simulink model "single_pend"  (R2019b)
settings: Solver=VariableStepAuto  StartTime=0.0  StopTime=20  RelTol=1e-3
values from neighbouring files (symbols this model uses):
  b = 200    [single_pend_runner.m]
  eta = 30.0    (= 30)    [single_pend_runner.m]
  g = 9.81    [G.m]    (also in connect_pend_runner.m = -9.81; run.m; single_pend_runner.m = -9.81)
  Kd = 50    [anujay_single_pendulum_same.m]    (also in connect_pend_runner.m; double_pend_setup.m = [50,0;0,50]; single_pend_runner.m = 500)
  Kp = 500    [single_pend_runner.m]
  l2 = l1    (= 1)    [connect_pend_runner.m]    (also in single_pend_runner.m = 3)
  lambda = 1.0    (= 1)    [single_pend_runner.m]
  m2 = 1.0 + m1    (= 2)    [connect_pend.m]    (also in connect_pend_runner.m; single_pend_runner.m = 10)
libraries: robotcorelib x1, simulink x1
settings Model: Creator=nathanielgoldfarb  LastModifiedBy=nathanielgoldfarb
settings SolverCC: ZeroCrossAlgorithm=Adaptive
settings DebuggingCC: IgnoredZcDiagnostic=none

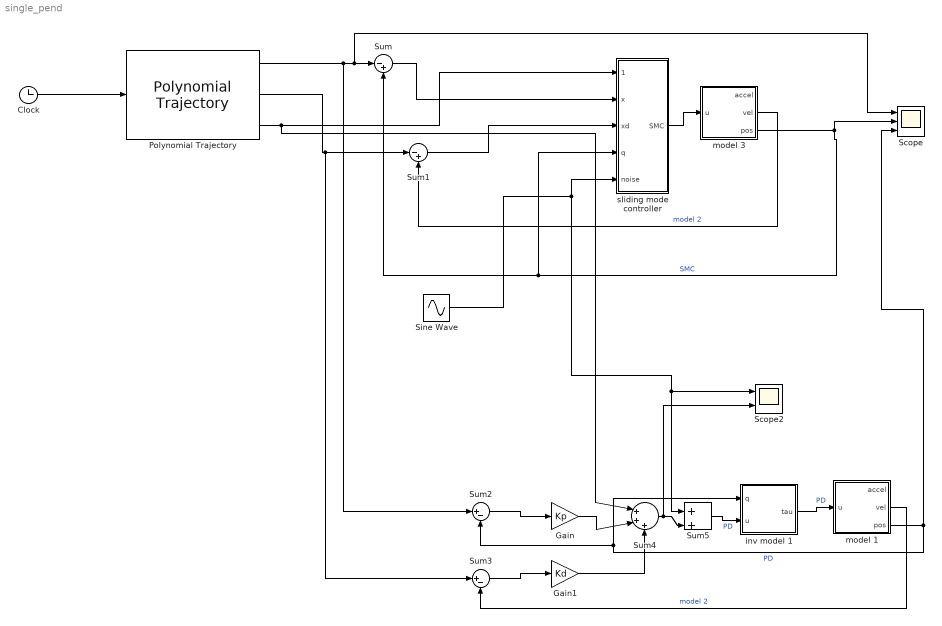
== system single_pend ==
  Clock : Clock
  Gain : Gain  Gain=Kp
  Gain1 : Gain  Gain=Kd
  Polynomial Trajectory : robotcorelib/Polynomial Trajectory  WaypointSource=Internal  Waypoints="[0  -pi ]"  TimePoints="[ 0,  5 ]"  TimeInterval=[ 1, 4 ]  Method=Cubic Polynomial  ParameterSource=Internal  VelocityBoundaryCondition=zeros( 1, 2 )  AccelerationBoundaryCondition=zeros( 2, 5 )  SimulateUsing=Interpreted execution
      settings: SourceProductName=Robotics System Toolbox  SourceProductBaseCode=RO
  Scope : Scope  NumInputPorts=3
  Scope2 : Scope  NumInputPorts=2
  Sine Wave : Sin  Amplitude=5  Frequency=50  SampleTime=0
  Sum : Sum  Inputs=|-+
  Sum1 : Sum  Inputs=|-+
  Sum2 : Sum  Inputs=|+-
  Sum3 : Sum  Inputs=|+-
  Sum4 : Sum  Inputs=|+++
  Sum5 : Sum  Inputs=|++
  inv model 1 : Subsystem
  model 1 : Subsystem
  model 3 : Subsystem
  sliding mode controller : Subsystem
  wires:
  Clock/1 -> Polynomial Trajectory/1
  sliding mode controller/1(SMC) -> model 3/1("u ")
  Polynomial Trajectory/3 -> Sum4/1, sliding mode controller/1(qdd desired)
  Polynomial Trajectory/1 -> Sum2/1, Scope/1, Sum/1
  model 3/3(pos) -> sliding mode controller/4(q), Sum/2, Scope/2  "SMC"
  Sum/1 -> sliding mode controller/2(x)
  Polynomial Trajectory/2 -> Sum3/1, Sum1/1
  model 3/2(vel) -> Sum1/2  "model 2"
  Sum1/1 -> sliding mode controller/3(xd)
  Sum2/1 -> Gain/1
  Sum3/1 -> Gain1/1
  model 1/3(pos) -> Scope/3, inv model 1/1(q), Sum2/2  "PD"
  model 1/2(vel) -> Sum3/2  "model 2"
  Gain1/1 -> Sum4/3
  Gain/1 -> Sum4/2
  inv model 1/1("tau ") -> model 1/1("u ")  "PD"
  Sum4/1 -> Scope2/2, Sum5/2
  Sum5/1 -> inv model 1/2("u ")  "PD"
  Sine Wave/1 -> sliding mode controller/5("noise "), Scope2/1, Sum5/1

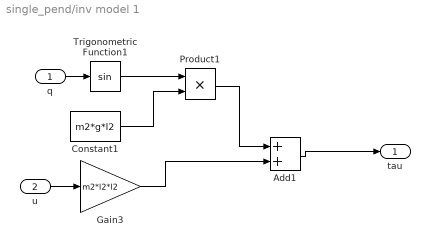
== system single_pend/inv model 1 ==
  q : Inport
  "u " : Inport  Port=2
  Add1 : Sum
  Constant1 : Constant  Value=m2*g*l2
  Gain3 : Gain  Gain=m2*l2*l2
  Product1 : Product
  Trigonometric Function1 : Trigonometry
  "tau " : Outport
  wires:
  Product1/1 -> Add1/1
  Constant1/1 -> Product1/2
  Add1/1 -> "tau "/1
  Gain3/1 -> Add1/2
  "u "/1 -> Gain3/1
  Trigonometric Function1/1 -> Product1/1
  q/1 -> Trigonometric Function1/1

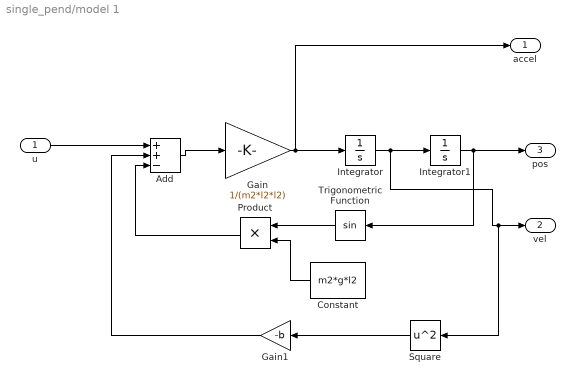
== system single_pend/model 1 ==
  "u " : Inport
  Add : Sum  Inputs=++-
  Constant : Constant  Value=m2*g*l2
  Gain : Gain  Gain=1/(m2*l2*l2)
  Gain1 : Gain  Gain=-b
  Integrator : Integrator
  Integrator1 : Integrator  InitialCondition=0.1
  Product : Product
  Square : Math  Operator=square  SignedPower=off  SaturateOnIntegerOverflow=on
  Trigonometric Function : Trigonometry
  accel : Outport
  vel : Outport  Port=2
  pos : Outport  Port=3
  wires:
  Trigonometric Function/1 -> Product/1
  Product/1 -> Add/3
  Add/1 -> Gain/1
  "u "/1 -> Add/1
  Gain/1 -> accel/1, Integrator/1
  Integrator/1 -> Square/1, vel/1, Integrator1/1
  Constant/1 -> Product/2
  Integrator1/1 -> pos/1, Trigonometric Function/1
  Gain1/1 -> Add/2
  Square/1 -> Gain1/1

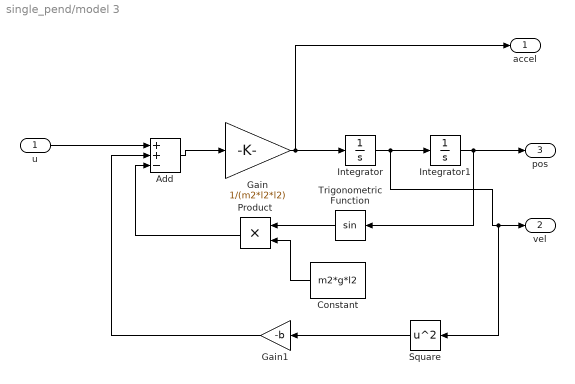
== system single_pend/model 3 ==
  "u " : Inport
  Add : Sum  Inputs=++-
  Constant : Constant  Value=m2*g*l2
  Gain : Gain  Gain=1/(m2*l2*l2)
  Gain1 : Gain  Gain=-b
  Integrator : Integrator
  Integrator1 : Integrator  InitialCondition=0.1
  Product : Product
  Square : Math  Operator=square  SignedPower=off  SaturateOnIntegerOverflow=on
  Trigonometric Function : Trigonometry
  accel : Outport
  vel : Outport  Port=2
  pos : Outport  Port=3
  wires:
  Trigonometric Function/1 -> Product/1
  Product/1 -> Add/3
  Add/1 -> Gain/1
  "u "/1 -> Add/1
  Gain/1 -> accel/1, Integrator/1
  Integrator/1 -> Square/1, vel/1, Integrator1/1
  Constant/1 -> Product/2
  Integrator1/1 -> pos/1, Trigonometric Function/1
  Gain1/1 -> Add/2
  Square/1 -> Gain1/1

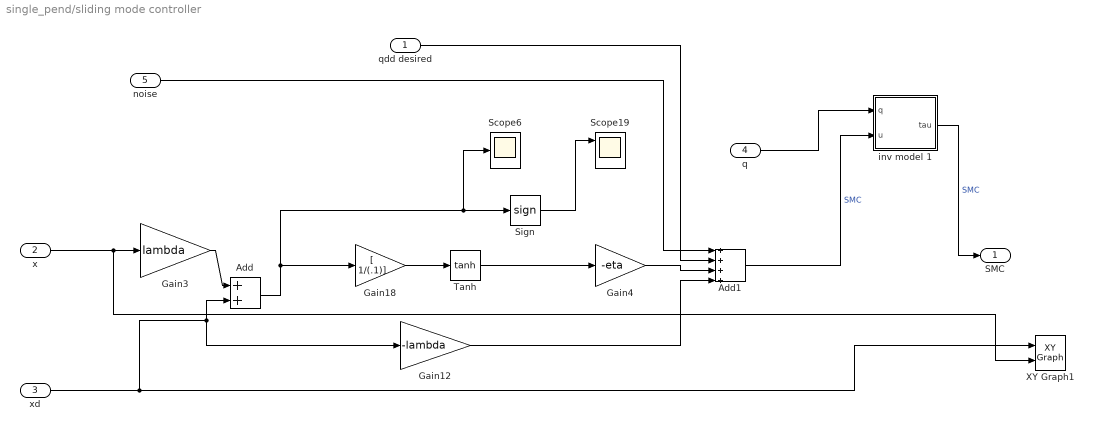
== system single_pend/sliding mode controller ==
  qdd desired : Inport
  x : Inport  Port=2
  xd : Inport  Port=3
  q : Inport  Port=4
  "noise " : Inport  Port=5
  Add : Sum
  Add1 : Sum  Inputs=++++
  Gain12 : Gain  Gain=-lambda
  Gain18 : Gain  Gain=[ 1/(.1)]
  Gain3 : Gain  Gain=lambda
  Gain4 : Gain  Gain=-eta
  Scope19 : Scope  NumInputPorts=2
  Scope6 : Scope
  Sign : Signum
  Tanh : Trigonometry  Operator=tanh
  XY Graph1 : simulink/Sinks/XY Graph  xmin=-0.1  xmax=0.1  ymin=-0.1  ymax=0.3  st=-1
  inv model 1 : Subsystem
  SMC : Outport
  wires:
  Gain12/1 -> Add1/4
  Gain3/1 -> Add/1
  q/1 -> inv model 1/1(q)
  x/1 -> XY Graph1/2, Gain3/1
  xd/1 -> XY Graph1/1, Add/2, Gain12/1
  Add/1 -> Scope6/1, Sign/1, Gain18/1
  Sign/1 -> Scope19/1
  Gain4/1 -> Add1/3
  qdd desired/1 -> Add1/2
  "noise "/1 -> Add1/1
  Gain18/1 -> Tanh/1
  Add1/1 -> inv model 1/2("u ")  "SMC"
  inv model 1/1("tau ") -> SMC/1  "SMC"
  Tanh/1 -> Gain4/1

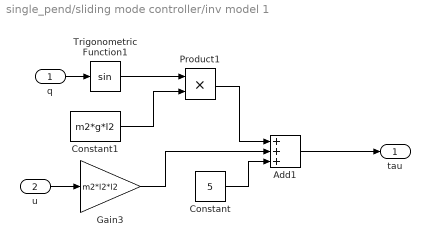
== system single_pend/sliding mode controller/inv model 1 ==
  q : Inport
  "u " : Inport  Port=2
  Add1 : Sum  Inputs=+++
  Constant : Constant  Value=5
  Constant1 : Constant  Value=m2*g*l2
  Gain3 : Gain  Gain=m2*l2*l2
  Product1 : Product
  Trigonometric Function1 : Trigonometry
  "tau " : Outport
  wires:
  Product1/1 -> Add1/1
  Constant1/1 -> Product1/2
  Add1/1 -> "tau "/1
  Gain3/1 -> Add1/2
  "u "/1 -> Gain3/1
  Trigonometric Function1/1 -> Product1/1
  q/1 -> Trigonometric Function1/1
  Constant/1 -> Add1/3
